simulink model "b6_formation"  (R2021b)
settings: Solver=FixedStepAuto  StartTime=0.0  StopTime=inf  FixedStep=sampleTime  RelTol=1e-3
PreLoadFcn:
  | % Simulation parameters
  | %load exampleMap
  | 
  | % Lidar parameters
  | sensorOffset = [0,0];
  | scanAngles = -pi/2:pi/6:pi/2;
  | maxRange = 0.3;
InitFcn:
  | sampleTime = 0.05;
  | nMedianSize=3;
  | % Robot parameters
  | wheelRadius = 0.0335;
  | robotRadius = 0.116/2;
  | 
  | %角速度坐标
  | ks=1;
  | 
  | % Lidar parameters
  | sensorOffset = [0,0];
  | scanAngles = -pi:pi/36:pi;
  | maxRange = 0.2;
  | 
  | %车初始位置
  | init_pose_1=[1  1.3  pi/2]';
  | init_pose_2=[0.85 1  pi/2]';
  | init_pose_3=[1.15 1  pi/2]';
  | init_pose_4=[0.7  0.7 pi/2]';
  | init_pose_5=[1  0.7 pi/2]';
  | init_pose_6=[1.3 0.7  pi/2]';
  | 
  | %pp算法性能参数
  | Vd_pp=0.2;
  | Wd_pp=pi;
  | dist_pp=0.2;
  | GoalRadius=0.1;
  | numSector=180;
  | rangeDis=[0.1,maxRange];
  | thresholds=[1/360 1/36];
  | safetyDis=0.2;
  | minimumTurningRadius=0.5*robotRadius;
  | recovery_w=0.05;
undefined symbols (not defined in the file): Angular, DiscIntNeverNeededParam, Linear, Pose, Twist
libraries: robotlib x42, dspstat3 x18, mobileRoboticsLib x7, robotmobilelib x6, robotalgslib x6
(part 5 of 5)

== matlab function b6_formation/Subsystem/Car Pose Listener4/Subsystem/sensor2vCar ==
  data: x_init output; y_init output; yaw_init output; flag output; poseNew input; poseMsg input
function [x_init,y_init,yaw_init,flag] = sensor2vCar(poseNew, poseMsg)
persistent x0 y0 yaw0 yaw1 x0_init y0_init yaw0_init fStart
if isempty(x0)
    x0=-10; y0=-10; yaw0=0; yaw1=0;   
    x0_init=-10;y0_init=-10;yaw0_init=0;
    fStart=0;
end
if poseNew
    if x0==poseMsg.Pose.Pose.Position.X&&y0==poseMsg.Pose.Pose.Position.Y
        flag=1;
    else
        x0=poseMsg.Pose.Pose.Position.X;
        y0=poseMsg.Pose.Pose.Position.Y;   
        %yaw2=atan2(2*(poseMsg.Pose.Pose.Orientation.Z*poseMsg.Pose.Pose.Orientation.W),1-2*(poseMsg.Pose.Pose.Orientation.Z^2)); 
        eul=quat2eul([poseMsg.Pose.Pose.Orientation.W,poseMsg.Pose.Pose.Orientation.X,poseMsg.Pose.Pose.Orientation.Y,poseMsg.Pose.Pose.Orientation.Z]);
        yaw2=eul(1);
        %对前后角度差使用积分，恢复yaw的连续性
        yaw0=yaw0+angdiff(yaw1,yaw2);
        yaw1=yaw2;
        flag=0;        
        x0_init=x0;
        y0_init=y0;
        yaw0_init=yaw0;
        fStart=1;
    end 
else
    if fStart
        flag=1;
    else
        flag=0;
    end
end

x_init=x0_init;y_init=y0_init;yaw_init=yaw0_init;

== matlab function b6_formation/Subsystem/Car Pose Listener4/Subsystem/sensor2vCar4 ==
  data: V output; W output; VW_New input; VW_Msg input
function [V,W] = sensor2vCar(VW_New, VW_Msg)
persistent v0 w0
if isempty(v0)
    v0=0; 
    w0=0;    
end
if VW_New
    v0=VW_Msg.Linear.X;
    w0=VW_Msg.Angular.Z;
end

V=v0;
W=-w0;

== matlab function b6_formation/Subsystem/Car Pose Listener5/Subsystem/sensor2vCar ==
  data: x_init output; y_init output; yaw_init output; flag output; poseNew input; poseMsg input
function [x_init,y_init,yaw_init,flag] = sensor2vCar(poseNew, poseMsg)
persistent x0 y0 yaw0 yaw1 x0_init y0_init yaw0_init fStart
if isempty(x0)
    x0=-10; y0=-10; yaw0=0; yaw1=0;   
    x0_init=-10;y0_init=-10;yaw0_init=0;
    fStart=0;
end
if poseNew
    if x0==poseMsg.Pose.Pose.Position.X&&y0==poseMsg.Pose.Pose.Position.Y
        flag=1;
    else
        x0=poseMsg.Pose.Pose.Position.X;
        y0=poseMsg.Pose.Pose.Position.Y;   
        %yaw2=atan2(2*(poseMsg.Pose.Pose.Orientation.Z*poseMsg.Pose.Pose.Orientation.W),1-2*(poseMsg.Pose.Pose.Orientation.Z^2)); 
        eul=quat2eul([poseMsg.Pose.Pose.Orientation.W,poseMsg.Pose.Pose.Orientation.X,poseMsg.Pose.Pose.Orientation.Y,poseMsg.Pose.Pose.Orientation.Z]);
        yaw2=eul(1);
        %对前后角度差使用积分，恢复yaw的连续性
        yaw0=yaw0+angdiff(yaw1,yaw2);
        yaw1=yaw2;
        flag=0;        
        x0_init=x0;
        y0_init=y0;
        yaw0_init=yaw0;
        fStart=1;
    end 
else
    if fStart
        flag=1;
    else
        flag=0;
    end
end

x_init=x0_init;y_init=y0_init;yaw_init=yaw0_init;

== matlab function b6_formation/Subsystem/Car Pose Listener5/Subsystem/sensor2vCar4 ==
  data: V output; W output; VW_New input; VW_Msg input
function [V,W] = sensor2vCar(VW_New, VW_Msg)
persistent v0 w0
if isempty(v0)
    v0=0; 
    w0=0;    
end
if VW_New
    v0=VW_Msg.Linear.X;
    w0=VW_Msg.Angular.Z;
end

V=v0;
W=-w0;

== matlab function b6_formation/controller/controller1/MATLAB Function2 ==
  data: poses input; idx input; ranges output; maxRange parameter; scanAngles parameter; robotRadius parameter

function ranges = genLidarSensor(poses,idx, maxRange, scanAngles, robotRadius)
%模拟激光雷达计算地图中障碍物距离

%计算部分
map=occupancyMap(3,3,50);
num=length(poses(1,:));%机器人总数
worldOffset=[0.5,0.5];%将世界坐标系偏移进地图
safetyDis=maxRange;
poseX=[poses(1,:)+worldOffset(1);poses(2,:)+worldOffset(2);poses(3,:)];
% for i=[1:idx-1 idx+1:num]
%     if poseX(i,1)>=0&&poseX(i,1)<=3&&poseX(i,2)>=0&&poseX(i,2)<=3        
%         setOccupancy(map,poseX(1:2,i)',1);
%     end
% end
obstacles = poseX(1:2,[1:idx-1 idx+1:num])';
setOccupancy(map,obstacles,ones(length(obstacles),1));
inflate(map,robotRadius);

if poseX(1,idx)>=0&&poseX(1,idx)<=3&&poseX(2,idx)>=0&&poseX(2,idx)<=3 
    vehiclePose = poseX(:,idx)';
    intsectionPts = rayIntersection(map,vehiclePose,scanAngles,safetyDis,0.7);
    offsets=intsectionPts-ones(length(scanAngles),1)*vehiclePose(1:2);
    ranges = sqrt(sum(offsets.^2,2));    
else
    ranges = nan(length(scanAngles),1);   
end

== matlab function b6_formation/controller/controller1/MATLAB Function3 ==
  data: poses input; idx input; ranges output; maxRange parameter; scanAngles parameter; robotRadius parameter

function ranges = genLidarSensor(poses,idx, maxRange, scanAngles, robotRadius)
%模拟激光雷达计算地图中障碍物距离

%计算部分
map=occupancyMap(3,3,50);
num=length(poses(1,:));%机器人总数
worldOffset=[0.5,0.5];%将世界坐标系偏移进地图
safetyDis=maxRange;
poseX=[poses(1,:)+worldOffset(1);poses(2,:)+worldOffset(2);poses(3,:)];
% for i=[1:idx-1 idx+1:num]
%     if poseX(i,1)>=0&&poseX(i,1)<=3&&poseX(i,2)>=0&&poseX(i,2)<=3        
%         setOccupancy(map,poseX(1:2,i)',1);
%     end
% end
obstacles = poseX(1:2,[1:idx-1 idx+1:num])';
setOccupancy(map,obstacles,ones(length(obstacles),1));
inflate(map,robotRadius);

if poseX(1,idx)>=0&&poseX(1,idx)<=3&&poseX(2,idx)>=0&&poseX(2,idx)<=3 
    vehiclePose = poseX(:,idx)';
    intsectionPts = rayIntersection(map,vehiclePose,scanAngles,safetyDis,0.7);
    offsets=intsectionPts-ones(length(scanAngles),1)*vehiclePose(1:2);
    ranges = sqrt(sum(offsets.^2,2));    
else
    ranges = nan(length(scanAngles),1);   
end

== matlab function b6_formation/controller/controller1/MATLAB Function10 ==
  data: poses input; idx input; ranges output; maxRange parameter; scanAngles parameter; robotRadius parameter

function ranges = genLidarSensor(poses,idx, maxRange, scanAngles, robotRadius)
%模拟激光雷达计算地图中障碍物距离

%计算部分
map=occupancyMap(3,3,50);
num=length(poses(1,:));%机器人总数
worldOffset=[0.5,0.5];%将世界坐标系偏移进地图
safetyDis=maxRange;
poseX=[poses(1,:)+worldOffset(1);poses(2,:)+worldOffset(2);poses(3,:)];
% for i=[1:idx-1 idx+1:num]
%     if poseX(i,1)>=0&&poseX(i,1)<=3&&poseX(i,2)>=0&&poseX(i,2)<=3        
%         setOccupancy(map,poseX(1:2,i)',1);
%     end
% end
obstacles = poseX(1:2,[1:idx-1 idx+1:num])';
setOccupancy(map,obstacles,ones(length(obstacles),1));
inflate(map,robotRadius);

if poseX(1,idx)>=0&&poseX(1,idx)<=3&&poseX(2,idx)>=0&&poseX(2,idx)<=3 
    vehiclePose = poseX(:,idx)';
    intsectionPts = rayIntersection(map,vehiclePose,scanAngles,safetyDis,0.7);
    offsets=intsectionPts-ones(length(scanAngles),1)*vehiclePose(1:2);
    ranges = sqrt(sum(offsets.^2,2));    
else
    ranges = nan(length(scanAngles),1);   
end

== matlab function b6_formation/controller/controller1/MATLAB Function4 ==
  data: poses input; idx input; ranges output; maxRange parameter; scanAngles parameter; robotRadius parameter

function ranges = genLidarSensor(poses,idx, maxRange, scanAngles, robotRadius)
%模拟激光雷达计算地图中障碍物距离

%计算部分
map=occupancyMap(3,3,50);
num=length(poses(1,:));%机器人总数
worldOffset=[0.5,0.5];%将世界坐标系偏移进地图
safetyDis=maxRange;
poseX=[poses(1,:)+worldOffset(1);poses(2,:)+worldOffset(2);poses(3,:)];
% for i=[1:idx-1 idx+1:num]
%     if poseX(i,1)>=0&&poseX(i,1)<=3&&poseX(i,2)>=0&&poseX(i,2)<=3        
%         setOccupancy(map,poseX(1:2,i)',1);
%     end
% end
obstacles = poseX(1:2,[1:idx-1 idx+1:num])';
setOccupancy(map,obstacles,ones(length(obstacles),1));
inflate(map,robotRadius);

if poseX(1,idx)>=0&&poseX(1,idx)<=3&&poseX(2,idx)>=0&&poseX(2,idx)<=3 
    vehiclePose = poseX(:,idx)';
    intsectionPts = rayIntersection(map,vehiclePose,scanAngles,safetyDis,0.7);
    offsets=intsectionPts-ones(length(scanAngles),1)*vehiclePose(1:2);
    ranges = sqrt(sum(offsets.^2,2));    
else
    ranges = nan(length(scanAngles),1);   
end

== matlab function b6_formation/Subsystem/Car Pose Listener/Subsystem/sensor2vCar ==
  data: x_init output; y_init output; yaw_init output; flag output; poseNew input; poseMsg input
function [x_init,y_init,yaw_init,flag] = sensor2vCar(poseNew, poseMsg)
persistent x0 y0 yaw0 yaw1 x0_init y0_init yaw0_init fStart
if isempty(x0)
    x0=-10; y0=-10; yaw0=0; yaw1=0;   
    x0_init=-10;y0_init=-10;yaw0_init=0;
    fStart=0;
end
if poseNew
    if x0==poseMsg.Pose.Pose.Position.X&&y0==poseMsg.Pose.Pose.Position.Y
        flag=1;
    else
        x0=poseMsg.Pose.Pose.Position.X;
        y0=poseMsg.Pose.Pose.Position.Y;   
        %yaw2=atan2(2*(poseMsg.Pose.Pose.Orientation.Z*poseMsg.Pose.Pose.Orientation.W),1-2*(poseMsg.Pose.Pose.Orientation.Z^2)); 
        eul=quat2eul([poseMsg.Pose.Pose.Orientation.W,poseMsg.Pose.Pose.Orientation.X,poseMsg.Pose.Pose.Orientation.Y,poseMsg.Pose.Pose.Orientation.Z]);
        yaw2=eul(1);
        %对前后角度差使用积分，恢复yaw的连续性
        yaw0=yaw0+angdiff(yaw1,yaw2);
        yaw1=yaw2;
        flag=0;        
        x0_init=x0;
        y0_init=y0;
        yaw0_init=yaw0;
        fStart=1;
    end 
else
    if fStart
        flag=1;
    else
        flag=0;
    end
end

x_init=x0_init;y_init=y0_init;yaw_init=yaw0_init;

== matlab function b6_formation/Subsystem/Car Pose Listener1/Subsystem/sensor2vCar4 ==
  data: V output; W output; VW_New input; VW_Msg input
function [V,W] = sensor2vCar(VW_New, VW_Msg)
persistent v0 w0
if isempty(v0)
    v0=0; 
    w0=0;    
end
if VW_New
    v0=VW_Msg.Linear.X;
    w0=VW_Msg.Angular.Z;
end

V=v0;
W=-w0;

== matlab function b6_formation/Subsystem/Car Pose Listener2/Subsystem/sensor2vCar ==
  data: x_init output; y_init output; yaw_init output; flag output; poseNew input; poseMsg input
function [x_init,y_init,yaw_init,flag] = sensor2vCar(poseNew, poseMsg)
persistent x0 y0 yaw0 yaw1 x0_init y0_init yaw0_init fStart
if isempty(x0)
    x0=-10; y0=-10; yaw0=0; yaw1=0;   
    x0_init=-10;y0_init=-10;yaw0_init=0;
    fStart=0;
end
if poseNew
    if x0==poseMsg.Pose.Pose.Position.X&&y0==poseMsg.Pose.Pose.Position.Y
        flag=1;
    else
        x0=poseMsg.Pose.Pose.Position.X;
        y0=poseMsg.Pose.Pose.Position.Y;   
        %yaw2=atan2(2*(poseMsg.Pose.Pose.Orientation.Z*poseMsg.Pose.Pose.Orientation.W),1-2*(poseMsg.Pose.Pose.Orientation.Z^2)); 
        eul=quat2eul([poseMsg.Pose.Pose.Orientation.W,poseMsg.Pose.Pose.Orientation.X,poseMsg.Pose.Pose.Orientation.Y,poseMsg.Pose.Pose.Orientation.Z]);
        yaw2=eul(1);
        %对前后角度差使用积分，恢复yaw的连续性
        yaw0=yaw0+angdiff(yaw1,yaw2);
        yaw1=yaw2;
        flag=0;        
        x0_init=x0;
        y0_init=y0;
        yaw0_init=yaw0;
        fStart=1;
    end 
else
    if fStart
        flag=1;
    else
        flag=0;
    end
end

x_init=x0_init;y_init=y0_init;yaw_init=yaw0_init;

== matlab function b6_formation/Subsystem/Car Pose Listener2/Subsystem/sensor2vCar4 ==
  data: V output; W output; VW_New input; VW_Msg input
function [V,W] = sensor2vCar(VW_New, VW_Msg)
persistent v0 w0
if isempty(v0)
    v0=0; 
    w0=0;    
end
if VW_New
    v0=VW_Msg.Linear.X;
    w0=VW_Msg.Angular.Z;
end

V=v0;
W=-w0;
